simulink library "CM340A_AdcDiagc_Library"  (R2013b)
settings: Solver=ode45  StartTime=0.0  StopTime=10.0  RelTol=1e-3
values from neighbouring files (symbols this model uses):
  ADCDIAGACCRCYFLTPRM_CNT_U08 = DataDict.Constant    [CM340A_AdcDiagc_DataDict.m]
  ADCDIAGCVLTGTHD_VOLT_F32 = DataDict.Constant    [CM340A_AdcDiagc_DataDict.m]
  ADCDIAGZEROFLTPRM_CNT_U08 = DataDict.Constant    [CM340A_AdcDiagc_DataDict.m]
  ARCHGLBPRM_FLOATZEROTHD_ULS_F32 = DataDict.Constant    [CM340A_AdcDiagc_DataDict.m]
libraries: simulink x1, CM340A_AdcDiagc_Library x1
settings Model: Creator=nz3zln  LastModifiedBy=wzvp6q

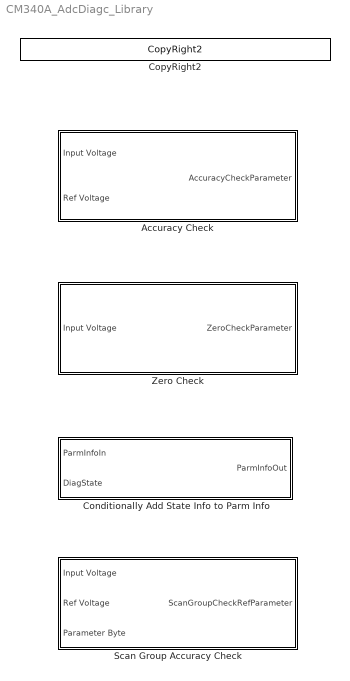
== system CM340A_AdcDiagc_Library ==
  Accuracy Check : Subsystem  TreatAsAtomicUnit=on
  Conditionally Add State Info to Parm Info : Subsystem  TreatAsAtomicUnit=on
  CopyRight2 : CM340A_AdcDiagc_Library/Scan Group Accuracy Check/CopyRight2  Description=|  none=on
      | Copyright info block.                                               
      |                                                                     
      | Place copyright information at the top of every subsystem in design.
  Scan Group Accuracy Check : Subsystem  TreatAsAtomicUnit=on
  Zero Check : Subsystem  TreatAsAtomicUnit=on

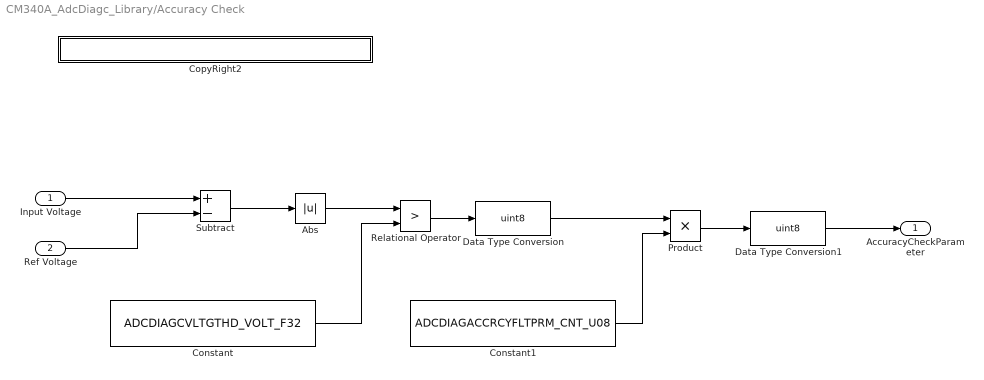
== system CM340A_AdcDiagc_Library/Accuracy Check ==
  Input Voltage : Inport  OutDataTypeStr=single
  Ref Voltage : Inport  Port=2  OutDataTypeStr=single
  Abs : Abs
  Constant : Constant  Value=ADCDIAGCVLTGTHD_VOLT_F32
  Constant1 : Constant  Value=ADCDIAGACCRCYFLTPRM_CNT_U08
  CopyRight2 : Subsystem  Description=|  mask(Copyright Information){none=on}
      | Copyright info block.                                               
      |                                                                     
      | Place copyright information at the top of every subsystem in design.
      mask prompts: none "No parameters"
      mask help: Place copyright information at the top of every subsystem in design.
      mask Display:
      | NxtrConf = 'Nexteer Confidential';
      | 
      | sys = bdroot; %handle for the current model ("system")
      | first = get_param(sys,'Created');
      | first = first(end-3:end);  %year is last four digits
      | 
      | last = get_param(sys,'LastModifiedDate');
      | if isempty(last)
      |     last = datestr(now,'yyyy');
      | else
      |     last = last(end-3:end);
      | end
      | 
      | if strcmp(first,last)
      |     fprintf('%s -- Copyright %s Nexteer',NxtrConf,first)
      | else
      |     fprintf('%s -- %s%s- %s Nexteer',NxtrConf,char(169),first,last)
      | end
  Data Type Conversion : DataTypeConversion  OutDataTypeStr=uint8
  Data Type Conversion1 : DataTypeConversion  OutDataTypeStr=uint8
  Product : Product
  Relational Operator : RelationalOperator  Operator=>  OutDataTypeStr=boolean
  Subtract : Sum  Inputs=+-
  AccuracyCheckParameter : Outport
  wires:
  Input Voltage/1 -> Subtract/1
  Ref Voltage/1 -> Subtract/2
  Subtract/1 -> Abs/1
  Abs/1 -> Relational Operator/1
  Constant/1 -> Relational Operator/2
  Relational Operator/1 -> Data Type Conversion/1
  Data Type Conversion/1 -> Product/1
  Constant1/1 -> Product/2
  Product/1 -> Data Type Conversion1/1
  Data Type Conversion1/1 -> AccuracyCheckParameter/1

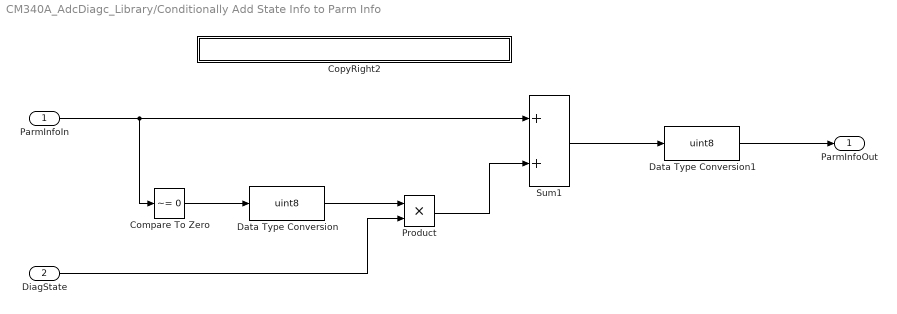
== system CM340A_AdcDiagc_Library/Conditionally Add State Info to Parm Info ==
  ParmInfoIn : Inport
  DiagState : Inport  Port=2
  Compare To Zero : simulink/Logic and Bit Operations/Compare To Zero  relop=~=  OutDataTypeStr=boolean
  CopyRight2 : Subsystem  Description=|  mask(Copyright Information){none=on}
      | Copyright info block.                                               
      |                                                                     
      | Place copyright information at the top of every subsystem in design.
      mask prompts: none "No parameters"
      mask help: Place copyright information at the top of every subsystem in design.
      mask Display:
      | NxtrConf = 'Nexteer Confidential';
      | 
      | sys = bdroot; %handle for the current model ("system")
      | first = get_param(sys,'Created');
      | first = first(end-3:end);  %year is last four digits
      | 
      | last = get_param(sys,'LastModifiedDate');
      | if isempty(last)
      |     last = datestr(now,'yyyy');
      | else
      |     last = last(end-3:end);
      | end
      | 
      | if strcmp(first,last)
      |     fprintf('%s -- Copyright %s Nexteer',NxtrConf,first)
      | else
      |     fprintf('%s -- %s%s- %s Nexteer',NxtrConf,char(169),first,last)
      | end
  Data Type Conversion : DataTypeConversion  OutDataTypeStr=uint8
  Data Type Conversion1 : DataTypeConversion  OutDataTypeStr=uint8
  Product : Product
  Sum1 : Sum
  ParmInfoOut : Outport
  wires:
  Product/1 -> Sum1/2
  DiagState/1 -> Product/2
  Data Type Conversion/1 -> Product/1
  Compare To Zero/1 -> Data Type Conversion/1
  ParmInfoIn/1 -> Sum1/1, Compare To Zero/1
  Sum1/1 -> Data Type Conversion1/1
  Data Type Conversion1/1 -> ParmInfoOut/1

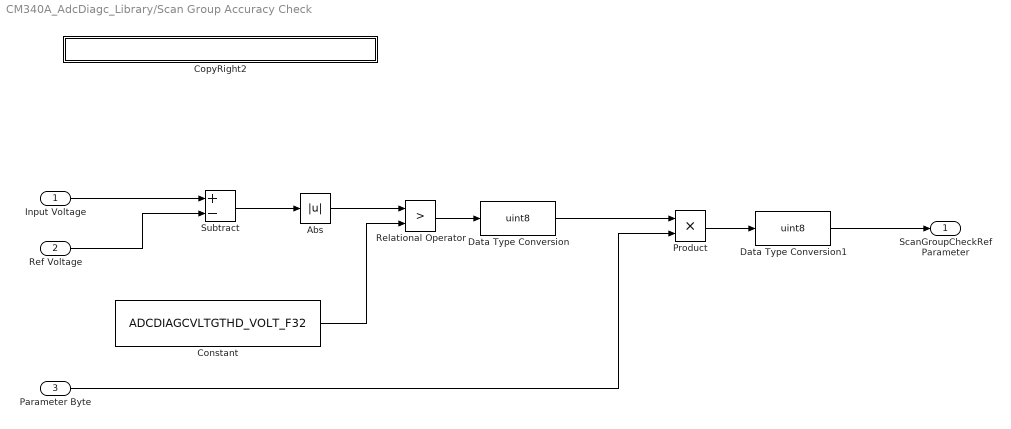
== system CM340A_AdcDiagc_Library/Scan Group Accuracy Check ==
  Input Voltage : Inport  OutDataTypeStr=single
  Ref Voltage : Inport  Port=2  OutDataTypeStr=single
  Parameter Byte : Inport  Port=3  OutDataTypeStr=uint8
  Abs : Abs
  Constant : Constant  Value=ADCDIAGCVLTGTHD_VOLT_F32
  CopyRight2 : Subsystem  Description=|  mask(Copyright Information){none=on}
      | Copyright info block.                                               
      |                                                                     
      | Place copyright information at the top of every subsystem in design.
      mask prompts: none "No parameters"
      mask help: Place copyright information at the top of every subsystem in design.
      mask Display:
      | NxtrConf = 'Nexteer Confidential';
      | 
      | sys = bdroot; %handle for the current model ("system")
      | first = get_param(sys,'Created');
      | first = first(end-3:end);  %year is last four digits
      | 
      | last = get_param(sys,'LastModifiedDate');
      | if isempty(last)
      |     last = datestr(now,'yyyy');
      | else
      |     last = last(end-3:end);
      | end
      | 
      | if strcmp(first,last)
      |     fprintf('%s -- Copyright %s Nexteer',NxtrConf,first)
      | else
      |     fprintf('%s -- %s%s- %s Nexteer',NxtrConf,char(169),first,last)
      | end
  Data Type Conversion : DataTypeConversion  OutDataTypeStr=uint8
  Data Type Conversion1 : DataTypeConversion  OutDataTypeStr=uint8
  Product : Product
  Relational Operator : RelationalOperator  Operator=>  OutDataTypeStr=boolean
  Subtract : Sum  Inputs=+-
  ScanGroupCheckRefParameter : Outport
  wires:
  Input Voltage/1 -> Subtract/1
  Ref Voltage/1 -> Subtract/2
  Subtract/1 -> Abs/1
  Abs/1 -> Relational Operator/1
  Constant/1 -> Relational Operator/2
  Relational Operator/1 -> Data Type Conversion/1
  Data Type Conversion/1 -> Product/1
  Parameter Byte/1 -> Product/2
  Product/1 -> Data Type Conversion1/1
  Data Type Conversion1/1 -> ScanGroupCheckRefParameter/1

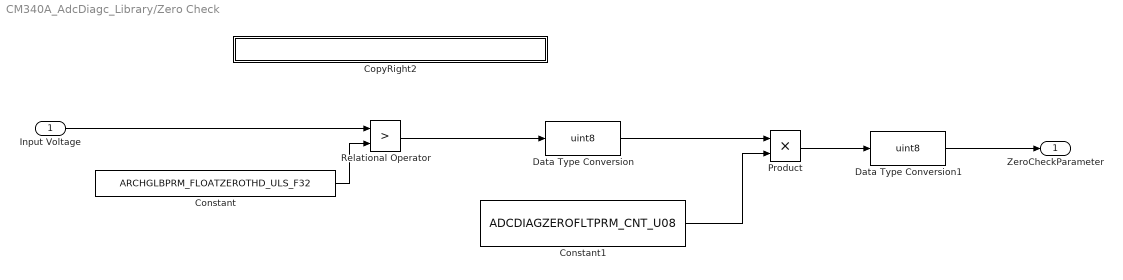
== system CM340A_AdcDiagc_Library/Zero Check ==
  Input Voltage : Inport  OutDataTypeStr=single
  Constant : Constant  Value=ARCHGLBPRM_FLOATZEROTHD_ULS_F32
  Constant1 : Constant  Value=ADCDIAGZEROFLTPRM_CNT_U08
  CopyRight2 : Subsystem  Description=|  mask(Copyright Information){none=on}
      | Copyright info block.                                               
      |                                                                     
      | Place copyright information at the top of every subsystem in design.
      mask prompts: none "No parameters"
      mask help: Place copyright information at the top of every subsystem in design.
      mask Display:
      | NxtrConf = 'Nexteer Confidential';
      | 
      | sys = bdroot; %handle for the current model ("system")
      | first = get_param(sys,'Created');
      | first = first(end-3:end);  %year is last four digits
      | 
      | last = get_param(sys,'LastModifiedDate');
      | if isempty(last)
      |     last = datestr(now,'yyyy');
      | else
      |     last = last(end-3:end);
      | end
      | 
      | if strcmp(first,last)
      |     fprintf('%s -- Copyright %s Nexteer',NxtrConf,first)
      | else
      |     fprintf('%s -- %s%s- %s Nexteer',NxtrConf,char(169),first,last)
      | end
  Data Type Conversion : DataTypeConversion  OutDataTypeStr=uint8
  Data Type Conversion1 : DataTypeConversion  OutDataTypeStr=uint8
  Product : Product
  Relational Operator : RelationalOperator  Operator=>  OutDataTypeStr=boolean
  ZeroCheckParameter : Outport
  wires:
  Input Voltage/1 -> Relational Operator/1
  Relational Operator/1 -> Data Type Conversion/1
  Data Type Conversion/1 -> Product/1
  Constant1/1 -> Product/2
  Product/1 -> Data Type Conversion1/1
  Data Type Conversion1/1 -> ZeroCheckParameter/1
  Constant/1 -> Relational Operator/2

== system CM340A_AdcDiagc_Library/Accuracy Check/CopyRight2 ==

== system CM340A_AdcDiagc_Library/Conditionally Add State Info to Parm Info/CopyRight2 ==

== system CM340A_AdcDiagc_Library/Scan Group Accuracy Check/CopyRight2 ==

== system CM340A_AdcDiagc_Library/Zero Check/CopyRight2 ==
